simulink model "Block"  (R2024b)
settings: Solver=VariableStepDiscrete  StartTime=0.0  StopTime=Inf  RelTol=1e-3
InitFcn:
  | InitFcn
values from neighbouring files (symbols this model uses):
  messageLength = 223    [InitFcn.m]    (also in TeoriaLab.m)
  ppoly = primpoly(m,'nodisplay')    [InitFcn.m]
  samplesPerFrame = lowerBound    [InitFcn.m]
libraries: commchan3 x4, commblkcod2 x4, commblkintrlv2 x4, commdigbbndam3 x4, commsink2 x2, commeq3 x2, dspstat3 x2, commrandsrc3 x1
settings Model: Creator=lukaszch  LastModifiedBy=jbojarczuk
settings SolverCC: AlgebraicLoopSolver=TrustRegion
settings DataIOCC: LimitDataPoints=on  SaveOutput=off  SignalLogging=off  DSMLogging=off  SaveTime=off  ReturnWorkspaceOutputs=off
settings OptimizationCC: BooleanDataType=off  DefaultParameterBehavior=Inlined  LocalBlockOutputs=off  LifeSpan=inf
settings DebuggingCC: ReadBeforeWriteMsg=DisableAll  WriteAfterWriteMsg=DisableAll  WriteAfterReadMsg=DisableAll  AlgebraicLoopMsg=error  MultiTaskDSMMsg=none  SingleTaskRateTransMsg=error  UnconnectedInputMsg=warning  UnconnectedOutputMsg=warning  UnconnectedLineMsg=warning  AllowSymbolicDim=off  SFUnexpectedBacktrackingDiag=warning  SFNoUnconditionalDefaultTransitionDiag=warning  SFExecutionAtInitializationDiag=none  ArithmeticOperatorsInVariantConditions=warning
settings ModelReferenceCC: UpdateModelReferenceTargets=IfOutOfDate  EnableRefExpFcnMdlSchedulingChecks=on
settings SFSimCC: SFSimEcho=off  SimUseLocalCustomCode=off  CustomCodeUndefinedFunction=UseInterfaceOnly
settings RTWCC: RTWUseLocalCustomCode=off  GPUComputeCapability=3.5
settings CodeAppCC: StateflowObjectComments=on
settings GRTTargetCC: TargetLangStandard=C89/C90 (ANSI)
settings ConfigComp: CovMetricSettings=dw  CovSaveCumulativeToWorkspaceVar=on  CovSaveSingleToWorkspaceVar=on  CovExternalEMLEnable=off  CovSFcnEnable=off

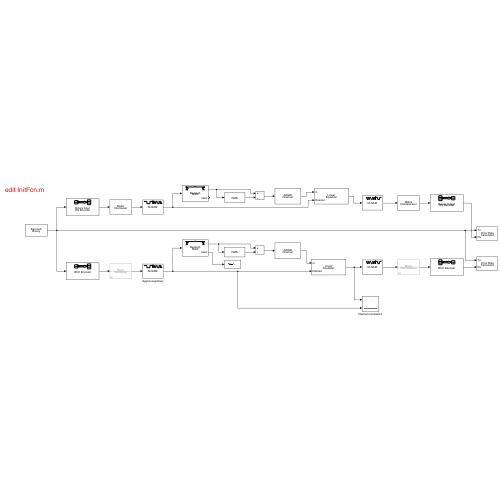
[thumbnail: Simulink's stored preview of the top-level diagram]
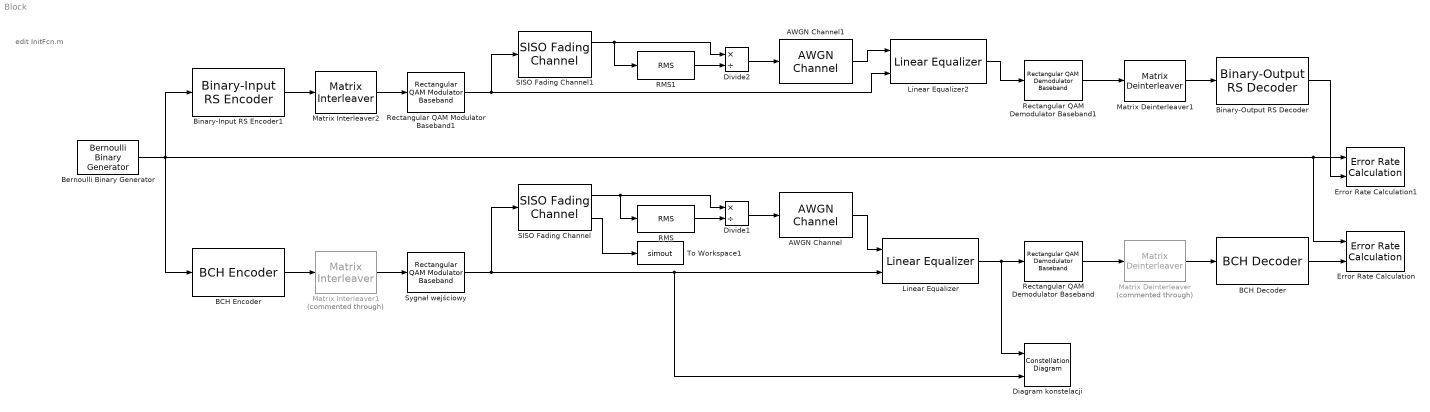
== system Block ==
  note: edit InitFcn.m
  AWGN Channel : commchan3/AWGN Channel  LegacyMode=on  NoiseMethod="Signal to noise ratio  (SNR)"  noiseMode="Signal to noise ratio  (SNR)"  EbNo=4  EsNo=10  SNR=snrAwgn  BitsPerSymbol=1  SignalPower=1  SamplesPerSymbol=1  SymbolPeriod=10  VarianceSource=Parameter  Variance=1  RandomStream=Global stream  Seed=67  SimulateUsing=Code generation
  AWGN Channel1 : commchan3/AWGN Channel  LegacyMode=on  NoiseMethod="Signal to noise ratio  (SNR)"  noiseMode="Signal to noise ratio  (SNR)"  EbNo=4  EsNo=10  SNR=snrAwgn  BitsPerSymbol=1  SignalPower=1  SamplesPerSymbol=1  SymbolPeriod=10  VarianceSource=Parameter  Variance=1  RandomStream=Global stream  Seed=67  SimulateUsing=Code generation
  BCH Decoder : commblkcod2/BCH Decoder  n=codewordLength  k=messageLength  specShortening=off  shortenedK=5  specGenPoly=on  genPoly=genPoly  specPrimPoly=on  prPoly=int2bit(ppoly,ceil(log2(max(ppoly))))'  specDisableGenCheck=on  specPuncture=off  punctVec=[ones(8,1); zeros(2,1)]  specErasurePort=off  showNumErr=off
  BCH Encoder : commblkcod2/BCH Encoder  n=codewordLength  k=messageLength  specShortening=off  shortenedK=5  specGenPoly=on  genPoly=genPoly  specPrimPoly=on  prPoly=int2bit(ppoly,ceil(log2(max(ppoly))))'  specDisableGenCheck=on  specPuncture=off  punctVec=[ones(8,1); zeros(2,1)]
  Bernoulli Binary Generator : commrandsrc3/Bernoulli Binary Generator  ProbabilityOfZero=0.5  SeedSource=Auto  Seed=0  SampleTime=1  SamplesPerFrame=samplesPerFrame  OutputDataType=double  SimulateUsing=Interpreted execution
  Binary-Input RS Encoder1 : commblkcod2/Binary-Input RS Encoder  n=codewordLength  k=messageLength  specShortening=off  shortenedK=3  specGenPoly=on  genPoly=genPolyRS  specPrimPoly=on  prPoly=int2bit(ppoly,ceil(log2(max(ppoly))))'  specPuncture=off  punctVec=[ones(2,1); zeros(2,1)]  outDType=Same as input
  Binary-Output RS Decoder : commblkcod2/Binary-Output RS Decoder  n=codewordLength  k=messageLength  specShortening=off  shortenedK=3  specGenPoly=on  genPoly=genPolyRS  specPrimPoly=on  prPoly=int2bit(ppoly,ceil(log2(max(ppoly))))'  specPuncture=off  punctVec=[ones(2,1); zeros(2,1)]  specErasurePort=off  showNumErr=off  outDType=Same as input
  Diagram konstelacji : ConstellationDiagram  NumInputPorts=2  WindowPosition=[1660.000000,515.000000,1413.000000,663.000000,]  Visible=on  ScopeFrameLocation=window  SymbolsToDisplaySource=Property  SymbolsToDisplay=8000  ReferenceConstellation={[QPSK][customReferenceConstellation]}  XLimits=[-3.78,4.39]  YLimits=[-1.46,1.96]  ShowLegend=on  ShowReferenceConstellation=off  DefaultConfigurationName=comm.scopes.ConstellationDiagramBlockCfg
  Divide1 : Product  Inputs=*/
  Divide2 : Product  Inputs=*/
  Error Rate Calculation : commsink2/Error Rate Calculation  N=0  st_delay=0  cp_mode=Entire frame  subframe=[]  PMode=Workspace  WsName=bchErr  RsMode2=off  stop=on  numErr=targetErr  maxBits=maxSymb
  Error Rate Calculation1 : commsink2/Error Rate Calculation  N=0  st_delay=0  cp_mode=Entire frame  subframe=[]  PMode=Workspace  WsName=rsErr  RsMode2=off  stop=on  numErr=targetErr  maxBits=maxSymb
  Linear Equalizer : commeq3/Linear Equalizer  NumTaps=eq.taps  Constellation=eq.const  InputSamplesPerSymbol=eq.sps  Algorithm=RLS  StepSize=0.01  ForgettingFactor=eq.lambda  InitialInverseCorrelationMatrix=0.1  ReferenceTap=eq.refTap  InputDelay=eq.inputDelay  AdaptWeightsSource=Property  AdaptWeights=on  InitialWeightsSource=Auto  InitialWeights=0  TrainingInitialWeights=0  BlindInitialWeights=[ 0; 0; 1; 0; 0 ]  WeightUpdatePeriod=eq.wUpdatePer  TrainingFlagInputPort=off  AdaptAfterTraining=off  ResetInputPort=off  ErrorOutputPort=off  TapWeightsOutputPort=off  SimulateUsing=Code generation
  Linear Equalizer2 : commeq3/Linear Equalizer  NumTaps=eq.taps  Constellation=eq.const  InputSamplesPerSymbol=eq.sps  Algorithm=RLS  StepSize=0.01  ForgettingFactor=eq.lambda  InitialInverseCorrelationMatrix=0.1  ReferenceTap=eq.refTap  InputDelay=eq.inputDelay  AdaptWeightsSource=Property  AdaptWeights=on  InitialWeightsSource=Auto  InitialWeights=0  TrainingInitialWeights=0  BlindInitialWeights=[ 0; 0; 1; 0; 0 ]  WeightUpdatePeriod=eq.wUpdatePer  TrainingFlagInputPort=off  AdaptAfterTraining=off  ResetInputPort=off  ErrorOutputPort=off  TapWeightsOutputPort=off  SimulateUsing=Code generation
  Matrix Deinterleaver : commblkintrlv2/Matrix Deinterleaver  Commented=through  StatePerturbationForJacobian=1.0e-05  Nrows=codewordLength  Ncols=samplesPerFrame/messageLength
  Matrix Deinterleaver1 : commblkintrlv2/Matrix Deinterleaver  StatePerturbationForJacobian=1.0e-05  Nrows=codewordLength  Ncols=samplesPerFrame/messageLength
  Matrix Interleaver1 : commblkintrlv2/Matrix Interleaver  Commented=through  StatePerturbationForJacobian=1.0e-05  Nrows=codewordLength  Ncols=samplesPerFrame/messageLength
  Matrix Interleaver2 : commblkintrlv2/Matrix Interleaver  StatePerturbationForJacobian=1.0e-05  Nrows=codewordLength  Ncols=samplesPerFrame/messageLength
  RMS : dspstat3/RMS  run=off  directionMode=Entire input  dimension=1  InputProcessing=Columns as channels (frame based)  reset_popup=None
  RMS1 : dspstat3/RMS  run=off  directionMode=Entire input  dimension=1  InputProcessing=Columns as channels (frame based)  reset_popup=None
  Rectangular QAM Demodulator Baseband : commdigbbndam3/Rectangular QAM Demodulator Baseband  M=Mary  OutType=Bit  DecType=Hard decision  VarSource=Dialog  Variance=1  Dec=Gray  Mapping=[0:15]  PowType=Average Power  MinDist=2  AvgPow=1  PeakPow=1  Ph=0  outDtype1=Inherit via internal rule  outDtype2=Inherit via internal rule  derotateFactorWordLen=16  derotateFactorDataTypeStr=Inherit: Same word length as input  derotateFactorLastDataTypeStr=Inherit: Same word length as input  denormFactorWordLen=16  denormFactorDataTypeStr=Inherit: Same word length as input  denormFactorLastDataTypeStr=Inherit: Same word length as input  prodOutWordLen=32  prodOutOverflowMode=Wrap  prodOutRoundingMode=Floor  prodOutOvFlMode=off  prodOutOvFlModeLastStrValue=off  sumWordLen=32
  Rectangular QAM Demodulator Baseband1 : commdigbbndam3/Rectangular QAM Demodulator Baseband  M=Mary  OutType=Bit  DecType=Hard decision  VarSource=Dialog  Variance=1  Dec=Gray  Mapping=[0:15]  PowType=Average Power  MinDist=2  AvgPow=1  PeakPow=1  Ph=0  outDtype1=Inherit via internal rule  outDtype2=Inherit via internal rule  derotateFactorWordLen=16  derotateFactorDataTypeStr=Inherit: Same word length as input  derotateFactorLastDataTypeStr=Inherit: Same word length as input  denormFactorWordLen=16  denormFactorDataTypeStr=Inherit: Same word length as input  denormFactorLastDataTypeStr=Inherit: Same word length as input  prodOutWordLen=32  prodOutOverflowMode=Wrap  prodOutRoundingMode=Floor  prodOutOvFlMode=off  prodOutOvFlModeLastStrValue=off  sumWordLen=32
  Rectangular QAM Modulator Baseband1 : commdigbbndam3/Rectangular QAM Modulator Baseband  M=Mary  InType=Bit  Enc=Gray  Mapping=[0:15]  PowType=Average Power  MinDist=2  AvgPow=1  PeakPow=1  Ph=0  outDtype=double  outWordLen=16  outUDDataType=sfix(16)  outFracLenMode=Best precision  outFracLen=15  outDataTypeStr=double  outLastDataTypeStr=double
  SISO Fading Channel : commchan3/SISO Fading Channel  InheritSampleRate=on  SampleRate=1  PathDelays=pathDelays  AveragePathGains=pathGains  NormalizePathGains=on  FadingDistribution=Rayleigh  KFactor=2  DirectPathDopplerShift=1e-7  DirectPathInitialPhase=0  MaximumDopplerShift=dopplerShift  DopplerSpectrum=dopplerSpectrum  RandomStream=mt19937ar with seed  Seed=73  PathGainsOutputPort=on  ChannelFilterDelayOutputPort=off  SimulateUsing=Interpreted execution  Visualization=Off  PathsForDopplerDisplay=1  SamplesToDisplay=25%
  SISO Fading Channel1 : commchan3/SISO Fading Channel  InheritSampleRate=on  SampleRate=1  PathDelays=pathDelays  AveragePathGains=pathGains  NormalizePathGains=on  FadingDistribution=Rayleigh  KFactor=3  DirectPathDopplerShift=0  DirectPathInitialPhase=0  MaximumDopplerShift=dopplerShift  DopplerSpectrum=dopplerSpectrum  RandomStream=mt19937ar with seed  Seed=73  PathGainsOutputPort=on  ChannelFilterDelayOutputPort=off  SimulateUsing=Interpreted execution  Visualization=Off  PathsForDopplerDisplay=1  SamplesToDisplay=25%
  Sygnał wejściowy : commdigbbndam3/Rectangular QAM Modulator Baseband  M=Mary  InType=Bit  Enc=Gray  Mapping=[0:15]  PowType=Average Power  MinDist=2  AvgPow=1  PeakPow=1  Ph=0  outDtype=double  outWordLen=16  outUDDataType=sfix(16)  outFracLenMode=Best precision  outFracLen=15  outDataTypeStr=double  outLastDataTypeStr=double
  To Workspace1 : ToWorkspace  VariableName=simout  SampleTime=-1
      settings: MaxDataPoints=samplesPerFrame*100  Decimation=10  Save2DSignal=2-D array (concatenate along first dimension)
  wires:
  Binary-Input RS Encoder1/1 -> Matrix Interleaver2/1
  Binary-Output RS Decoder/1 -> Error Rate Calculation1/2
  Bernoulli Binary Generator/1 -> Error Rate Calculation/1, Error Rate Calculation1/1, BCH Encoder/1, Binary-Input RS Encoder1/1
  AWGN Channel1/1 -> Linear Equalizer2/1
  BCH Encoder/1 -> Matrix Interleaver1/1
  RMS/1 -> Divide1/2
  Matrix Interleaver1/1 -> Sygnał wejściowy/1
  Matrix Interleaver2/1 -> Rectangular QAM Modulator Baseband1/1
  SISO Fading Channel/1 -> Divide1/1, RMS/1
  Sygnał wejściowy/1 -> Diagram konstelacji/2, Linear Equalizer/2, SISO Fading Channel/1
  SISO Fading Channel1/1 -> RMS1/1, Divide2/1
  SISO Fading Channel/2 -> To Workspace1/1
  Rectangular QAM Modulator Baseband1/1 -> Linear Equalizer2/2, SISO Fading Channel1/1
  Rectangular QAM Demodulator Baseband1/1 -> Matrix Deinterleaver1/1
  RMS1/1 -> Divide2/2
  Divide1/1 -> AWGN Channel/1
  Divide2/1 -> AWGN Channel1/1
  AWGN Channel/1 -> Linear Equalizer/1
  Linear Equalizer2/1 -> Rectangular QAM Demodulator Baseband1/1
  Linear Equalizer/1 -> Diagram konstelacji/1, Rectangular QAM Demodulator Baseband/1
  Rectangular QAM Demodulator Baseband/1 -> Matrix Deinterleaver/1
  Matrix Deinterleaver1/1 -> Binary-Output RS Decoder/1
  Matrix Deinterleaver/1 -> BCH Decoder/1
  BCH Decoder/1 -> Error Rate Calculation/2
